simulink model "sampleModel2024"  (R2023a)
settings: Solver=VariableStepAuto  StartTime=0.0  StopTime=10.0  RelTol=1e-3
libraries: hdlsllib x2, simulink x1
settings Model: Creator=user1  LastModifiedBy=user1

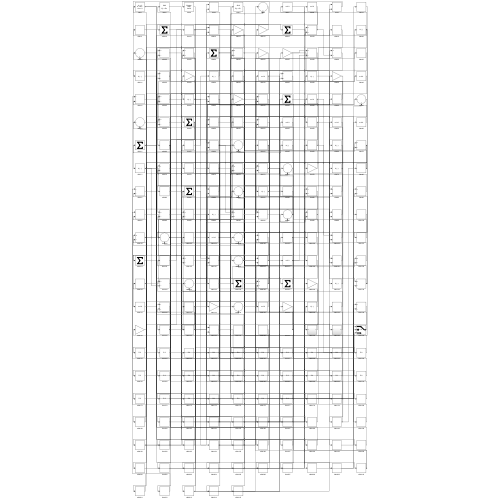
[thumbnail: Simulink's stored preview of the top-level diagram]
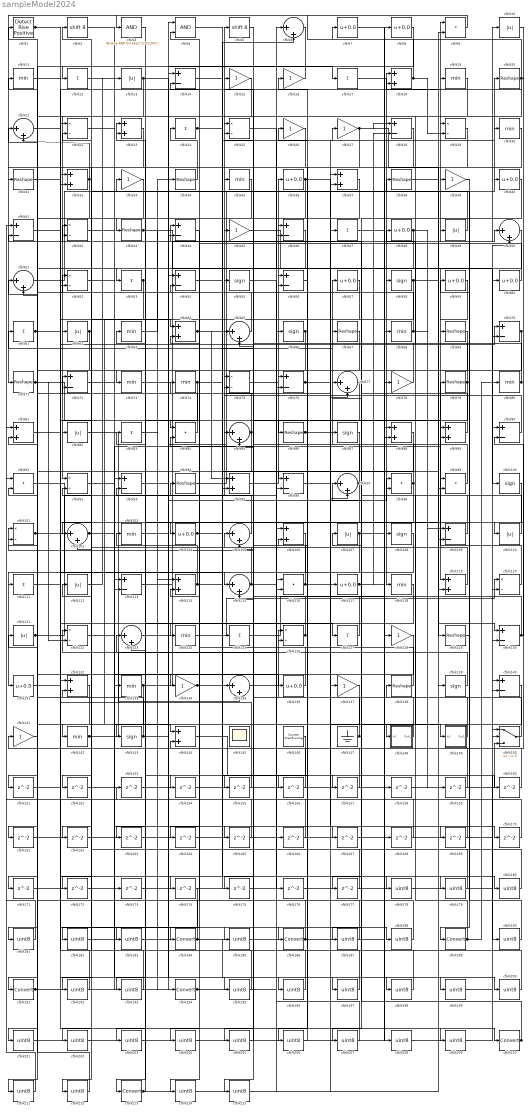
== system sampleModel2024 ==
  cfblk1 : hdlsllib/Logic and Bit Operations/Detect Rise Positive  vinit=0  OutDataTypeStr=boolean
  cfblk{10,13,49,62,82,107,110,112,121} (9 alike) : Abs  SaturateOnIntegerOverflow=off
  cfblk{55,58,66,87,100,108,139,143} (8 alike) : Signum
  cfblk{22,25,29,42,52,75,92,101,120,122,126} (11 alike) : Product  Inputs=*/  RndMeth=Zero  SaturateOnIntegerOverflow=on
  cfblk{6,21,50..51,65,77,85,97,102,105,115,123,135} (13 alike) : Sum  Inputs=|++
  cfblk{11,19,30,35,63,68,73..74,80,103,118,124,133,142} (14 alike) : MinMax
  cfblk{7..8,36,40,48,57,59..60,104,117,131,136} (12 alike) : Bias  Bias=0.0  SaturateOnIntegerOverflow=off
  cfblk{18,23,32,37,64,81,88..89,95,106,114,119,132,144} (14 alike) : Sum
  cfblk{14,28,41,44,46,54,56,70,72,76,90,93,96,109,113,130,140} (17 alike) : Sum  Inputs=+-
  cfblk{12,17,24,47,53,61,83,111,125,127} (10 alike) : Sum  Inputs=+
  cfblk{9,84,91,98..99,116} (6 alike) : DotProduct  OutDataTypeStr=Inherit: Inherit via internal rule
  cfblk{15..16,26..27,33,39,45,78,128,134,137,141} (12 alike) : Gain
  cfblk{20,31,34,38,43,67,69,71,79,86,94,129,138} (13 alike) : Reshape
  cfblk145 : Scope
      settings: Floating=on
  cfblk146 : hdlsllib/Sources/Counter Free-Running  NumBits=16  tsamp=-1
  cfblk147 : Ground
  cfblk148 : Subsystem
      settings: LibrarySourceBlock=|
      | hdlsllib/Ports &
      | Subsystems/Subsystem
  cfblk149 : Subsystem
      settings: LibrarySourceBlock=|
      | hdlsllib/Ports &
      | Subsystems/Subsystem
  cfblk150 : Switch  SaturateOnIntegerOverflow=off  InputSameDT=off
  cfblk{151..177} (27 alike) : Delay  SampleTime=1
  cfblk{178..183,185,187..188,190,192..193,195..209,211..212,214..215} (31 alike) : DataTypeConversion  OutDataTypeStr=uint8  SaturateOnIntegerOverflow=off  RndMeth=Floor
  cfblk{184,186,189,191,194,210,213} (7 alike) : DataTypeConversion  SaturateOnIntegerOverflow=off  RndMeth=Floor
  cfblk2 : ArithShift  BitShiftNumber=8
  cfblk3 : simulink/Logic and Bit Operations/Bitwise Operator  logicop=AND  UseBitMask=on  BitMask=bin2dec('11011001')  BitMaskRealWorld=Stored Integer
      settings: LibrarySourceBlock=|
      | hdlsllib/Logic and Bit
      | Operations/Bitwise
      | Operator
  cfblk4 : Logic  AllPortsSameDT=off  OutDataTypeStr=boolean
  cfblk5 : ArithShift  BitShiftNumber=8
  wires:
  cfblk34/1 -> cfblk24/1
  cfblk18/1 -> cfblk71/1, cfblk29/2
  cfblk95/1 -> cfblk36/1
  cfblk32/1 -> cfblk92/1, cfblk21/2
  cfblk112/1 -> cfblk13/1
  cfblk16/1 -> cfblk12/1
  cfblk20/1 -> cfblk62/1, cfblk7/1, cfblk110/1, cfblk18/2
  cfblk78/1 -> cfblk44/1
  cfblk9/1 -> cfblk3/1
  cfblk53/1 -> cfblk142/1, cfblk102/2
  cfblk17/1 -> cfblk118/1
  cfblk59/1 -> cfblk119/1
  cfblk63/1 -> cfblk34/1
  cfblk113/1 -> cfblk9/1
  cfblk82/1 -> cfblk135/2
  cfblk97/1 -> cfblk57/1, cfblk46/1, cfblk183/1
  cfblk109/1 -> cfblk56/1
  cfblk94/1 -> cfblk38/1
  cfblk121/1 -> cfblk5/1, cfblk101/1
  cfblk148/1(Out1) -> cfblk138/1
  cfblk36/1 -> cfblk51/2, cfblk170/1
  cfblk70/1 -> cfblk102/1, cfblk187/1
  cfblk71/1 -> cfblk89/1, cfblk122/2, cfblk197/1
  cfblk75/1 -> cfblk76/1
  cfblk49/1 -> cfblk2/1
  cfblk25/1 -> cfblk58/1
  cfblk150/1 -> cfblk25/1
  cfblk125/1 -> cfblk8/1
  cfblk118/1 -> cfblk123/2
  cfblk142/1 -> cfblk66/1, cfblk52/1
  cfblk51/1 -> cfblk20/1
  cfblk38/1 -> cfblk119/2
  cfblk147/1 -> cfblk126/1, cfblk101/2
  cfblk10/1 -> cfblk141/1
  cfblk133/1 -> cfblk10/1, cfblk182/1
  cfblk83/1 -> cfblk194/1
  cfblk73/1 -> cfblk49/1
  cfblk89/1 -> cfblk42/1
  cfblk80/1 -> cfblk48/1, cfblk73/1
  cfblk115/1 -> cfblk27/1, cfblk40/1, cfblk42/2
  cfblk139/1 -> cfblk122/1
  cfblk12/1 -> cfblk84/1
  cfblk135/1 -> cfblk126/2
  cfblk65/1 -> cfblk11/1
  cfblk132/1 -> cfblk191/1
  cfblk127/1 -> cfblk84/2
  cfblk68/1 -> cfblk45/1, cfblk109/1
  cfblk130/1 -> cfblk15/1, cfblk90/2
  cfblk5/1 -> cfblk115/1
  cfblk85/1 -> cfblk21/1, cfblk214/1
  cfblk43/1 -> cfblk69/1, cfblk114/1
  cfblk108/1 -> cfblk131/1
  cfblk64/1 -> cfblk95/1, cfblk109/2, cfblk169/1
  cfblk27/1 -> cfblk129/1, cfblk31/1, cfblk28/1
  cfblk54/1 -> cfblk50/1
  cfblk129/1 -> cfblk59/1
  cfblk134/1 -> cfblk18/1, cfblk64/2
  cfblk119/1 -> cfblk105/1
  cfblk3/1 -> cfblk43/1
  cfblk90/1 -> cfblk75/1
  cfblk99/1 -> cfblk72/1
  cfblk123/1 -> cfblk47/1
  cfblk92/1 -> cfblk124/1
  cfblk39/1 -> cfblk189/1
  cfblk66/1 -> cfblk111/1, cfblk175/1
  cfblk141/1 -> cfblk121/1
  cfblk124/1 -> cfblk120/1
  cfblk74/1 -> cfblk143/1, cfblk99/2
  cfblk1/1 -> cfblk108/1, cfblk185/1
  cfblk48/1 -> cfblk82/1, cfblk159/1
  cfblk76/1 -> cfblk97/2, cfblk77/2
  cfblk111/1 -> cfblk70/1
  cfblk84/1 -> cfblk33/1
  cfblk60/1 -> cfblk14/2
  cfblk107/1 -> cfblk116/2, cfblk180/1
  cfblk96/1 -> cfblk117/1
  cfblk114/1 -> cfblk23/1, cfblk157/1
  cfblk116/1 -> cfblk41/2, cfblk149/1(In1)
  cfblk149/1(Out1) -> cfblk56/2
  cfblk58/1 -> cfblk130/1, cfblk105/2
  cfblk81/1 -> cfblk210/1
  cfblk14/1 -> cfblk65/1
  cfblk131/1 -> cfblk32/2
  cfblk98/1 -> cfblk134/1, cfblk61/1
  cfblk29/1 -> cfblk44/2
  cfblk62/1 -> cfblk171/1, cfblk172/1
  cfblk44/1 -> cfblk104/1
  cfblk69/1 -> cfblk96/1
  cfblk126/1 -> cfblk94/1, cfblk85/2
  cfblk19/1 -> cfblk148/1(In1)
  cfblk79/1 -> cfblk35/1, cfblk215/1
  cfblk11/1 -> cfblk113/2
  cfblk102/1 -> cfblk144/1, cfblk89/2
  cfblk93/1 -> cfblk186/1
  cfblk77/1 -> cfblk115/2
  cfblk37/1 -> cfblk213/1
  cfblk2/1 -> cfblk136/1
  cfblk91/1 -> cfblk125/1
  cfblk45/1 -> cfblk100/1
  cfblk7/1 -> cfblk78/1
  cfblk13/1 -> cfblk17/1, cfblk52/2, cfblk167/1
  cfblk86/1 -> cfblk16/1, cfblk29/1
  cfblk87/1 -> cfblk184/1
  cfblk136/1 -> cfblk74/1
  cfblk120/1 -> cfblk79/1
  cfblk143/1 -> cfblk85/1, cfblk98/1, cfblk51/1
  cfblk104/1 -> cfblk30/1, cfblk67/1
  cfblk61/1 -> cfblk127/1, cfblk174/1
  cfblk138/1 -> cfblk25/2
  cfblk31/1 -> cfblk64/1
  cfblk117/1 -> cfblk28/2, cfblk209/1
  cfblk24/1 -> cfblk6/2, cfblk160/1
  cfblk21/1 -> cfblk86/1
  cfblk110/1 -> cfblk99/1
  cfblk8/1 -> cfblk53/1
  cfblk105/1 -> cfblk63/1
  cfblk101/1 -> cfblk6/1, cfblk19/1
  cfblk15/1 -> cfblk151/1
  cfblk57/1 -> cfblk152/1
  cfblk152/1 -> cfblk90/1
  cfblk153/1 -> cfblk150/3
  cfblk106/1 -> cfblk154/1
  cfblk154/1 -> cfblk76/2
  cfblk100/1 -> cfblk155/1
  cfblk155/1 -> cfblk32/1
  cfblk56/1 -> cfblk156/1
  cfblk156/1 -> cfblk113/1
  cfblk157/1 -> cfblk54/2
  cfblk158/1 -> cfblk150/2
  cfblk159/1 -> cfblk75/2
  cfblk160/1 -> cfblk65/2
  cfblk6/1 -> cfblk161/1
  cfblk161/1 -> cfblk135/1
  cfblk33/1 -> cfblk162/1
  cfblk162/1 -> cfblk70/2
  cfblk30/1 -> cfblk163/1
  cfblk163/1 -> cfblk14/1
  cfblk67/1 -> cfblk164/1
  cfblk164/1 -> cfblk96/2
  cfblk122/1 -> cfblk165/1
  cfblk165/1 -> cfblk41/1
  cfblk166/1 -> cfblk144/2
  cfblk47/1 -> cfblk168/1
  cfblk168/1 -> cfblk123/1
  cfblk169/1 -> cfblk97/1
  cfblk170/1 -> cfblk1/1
  cfblk171/1 -> cfblk130/2
  cfblk172/1 -> cfblk95/2
  cfblk72/1 -> cfblk173/1
  cfblk173/1 -> cfblk9/2
  cfblk175/1 -> cfblk120/2
  cfblk55/1 -> cfblk176/1
  cfblk176/1 -> cfblk50/2
  cfblk40/1 -> cfblk177/1
  cfblk177/1 -> cfblk92/2
  cfblk4/1 -> cfblk178/1
  cfblk178/1 -> cfblk60/1
  cfblk151/1 -> cfblk179/1
  cfblk179/1 -> cfblk4/1
  cfblk180/1 -> cfblk4/2
  cfblk88/1 -> cfblk181/1
  cfblk181/1 -> cfblk91/1
  cfblk182/1 -> cfblk88/1
  cfblk183/1 -> cfblk88/2
  cfblk184/1 -> cfblk72/2, cfblk91/2, cfblk198/1
  cfblk185/1 -> cfblk87/1
  cfblk186/1 -> cfblk114/2, cfblk68/1, cfblk106/2
  cfblk187/1 -> cfblk93/1
  cfblk52/1 -> cfblk188/1
  cfblk188/1 -> cfblk93/2
  cfblk189/1 -> cfblk98/2, cfblk80/1
  cfblk144/1 -> cfblk190/1
  cfblk190/1 -> cfblk39/1
  cfblk191/1 -> cfblk133/1, cfblk54/1
  cfblk35/1 -> cfblk192/1
  cfblk192/1 -> cfblk132/1
  cfblk146/1 -> cfblk193/1
  cfblk193/1 -> cfblk132/2
  cfblk194/1 -> cfblk46/2, cfblk106/1
  cfblk42/1 -> cfblk195/1
  cfblk195/1 -> cfblk83/1
  cfblk22/1 -> cfblk196/1
  cfblk196/1 -> cfblk112/1
  cfblk197/1 -> cfblk22/1
  cfblk198/1 -> cfblk22/2
  cfblk103/1 -> cfblk199/1
  cfblk199/1 -> cfblk150/1
  cfblk41/1 -> cfblk200/1
  cfblk200/1 -> cfblk103/1
  cfblk128/1 -> cfblk201/1
  cfblk201/1 -> cfblk158/1
  cfblk23/1 -> cfblk202/1
  cfblk202/1 -> cfblk128/1
  cfblk137/1 -> cfblk203/1
  cfblk203/1 -> cfblk153/1
  cfblk46/1 -> cfblk204/1
  cfblk204/1 -> cfblk137/1
  cfblk26/1 -> cfblk205/1
  cfblk205/1 -> cfblk55/1
  cfblk28/1 -> cfblk206/1
  cfblk206/1 -> cfblk26/1
  cfblk140/1 -> cfblk207/1
  cfblk207/1 -> cfblk116/1
  cfblk167/1 -> cfblk208/1
  cfblk208/1 -> cfblk140/1
  cfblk209/1 -> cfblk140/2
  cfblk210/1 -> cfblk77/1, cfblk107/1
  cfblk50/1 -> cfblk211/1
  cfblk211/1 -> cfblk81/1
  cfblk174/1 -> cfblk212/1
  cfblk212/1 -> cfblk81/2
  cfblk213/1 -> cfblk166/1, cfblk23/2, cfblk139/1
  cfblk214/1 -> cfblk37/1
  cfblk215/1 -> cfblk37/2

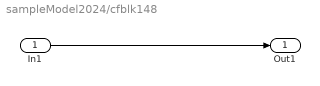
== system sampleModel2024/cfblk148 ==
  In1 : Inport
  Out1 : Outport
  wires:
  In1/1 -> Out1/1

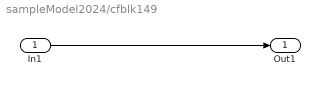
== system sampleModel2024/cfblk149 ==
  In1 : Inport
  Out1 : Outport
  wires:
  In1/1 -> Out1/1
